simulink model "HomeworkSimulink"  (R2020a)
settings: Solver=VariableStepAuto  StartTime=0.0  StopTime=10.0  RelTol=1e-3
libraries: simulink x1
settings Model: Creator=cresp  LastModifiedBy=cresp

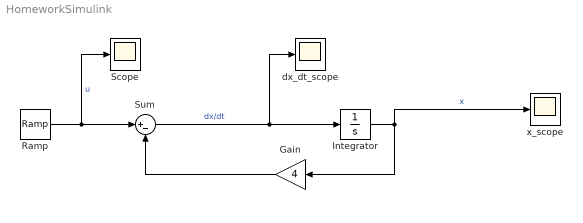
== system HomeworkSimulink ==
  Gain : Gain  Gain=4
  Integrator : Integrator
  Ramp : simulink/Sources/Ramp  slope=1  start=0  InitialOutput=0
  Scope : Scope
  Sum : Sum  Inputs=|+-
  dx_dt_scope : Scope
  x_scope : Scope
  wires:
  Sum/1 -> dx_dt_scope/1, Integrator/1  "dx/dt"
  Integrator/1 -> Gain/1, x_scope/1  "x"
  Gain/1 -> Sum/2
  Ramp/1 -> Scope/1, Sum/1  "u"
